simulink library "Byte_Multiplexers_Lib"  (Simulink 8.1)
settings: Solver=ode45  StartTime=0.0  StopTime=10.0  RelTol=1e-3
libraries: commutil2 x35, Bit_Multiplexers_Lib x32, Computer_Library x17
settings Model: Creator=uzivatel  LastModifiedBy=uzivatel

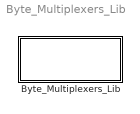
== system Byte_Multiplexers_Lib ==
  Byte_Multiplexers_Lib : Subsystem

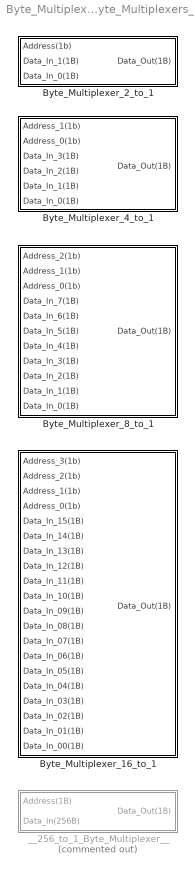
== system Byte_Multiplexers_Lib/Byte_Multiplexers_Lib ==
  Byte_Multiplexer_16_to_1 : Subsystem
  Byte_Multiplexer_2_to_1 : Subsystem
  Byte_Multiplexer_4_to_1 : Subsystem
  Byte_Multiplexer_8_to_1 : Subsystem
  __256_to_1_Byte_Multiplexer__ : Subsystem  Commented=on

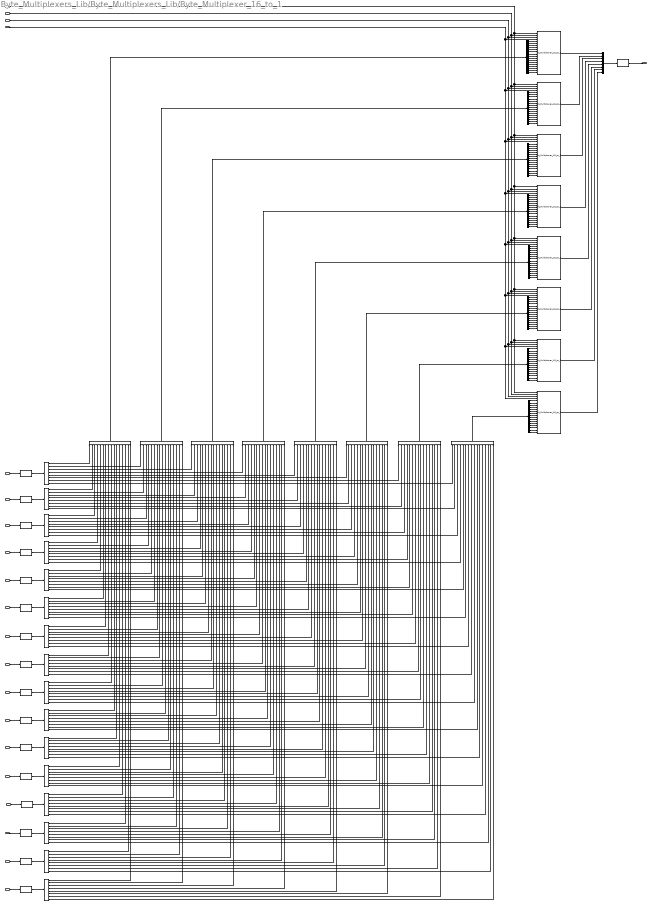
== system Byte_Multiplexers_Lib/Byte_Multiplexers_Lib/Byte_Multiplexer_16_to_1 ==
  Address_3(1b) : Inport
  Address_2(1b) : Inport  Port=2
  Address_1(1b) : Inport  Port=3
  Address_0(1b) : Inport  Port=4
  Data_In_15(1B) : Inport  Port=5
  Data_In_14(1B) : Inport  Port=6
  Data_In_13(1B) : Inport  Port=7
  Data_In_12(1B) : Inport  Port=8
  Data_In_11(1B) : Inport  Port=9
  Data_In_10(1B) : Inport  Port=10
  Data_In_09(1B) : Inport  Port=11
  Data_In_08(1B) : Inport  Port=12
  Data_In_07(1B) : Inport  Port=13
  Data_In_06(1B) : Inport  Port=14
  Data_In_05(1B) : Inport  Port=15
  Data_In_04(1B) : Inport  Port=16
  Data_In_03(1B) : Inport  Port=17
  Data_In_02(1B) : Inport  Port=18
  Data_In_01(1B) : Inport  Port=19
  Data_In_00(1B) : Inport  Port=20
  Bit to Integer Converter1 : commutil2/Bit to Integer Converter  nbits=8  bitOrder=MSB first  signedOutputValues=Unsigned  outDtype=uint8  outDtypeSigned=Inherit via internal rule
  Bit_{0..7} (8 alike) : Mux  Inputs=16
  Bit_Multiplexer_16_to_1(Bit_0) : Bit_Multiplexers_Lib/Bit_Multiplexers_Lib/Bit_Multiplexer_16_to_1
  Bit_Multiplexer_16_to_1(Bit_1) : Bit_Multiplexers_Lib/Bit_Multiplexers_Lib/Bit_Multiplexer_16_to_1
  Bit_Multiplexer_16_to_1(Bit_2) : Bit_Multiplexers_Lib/Bit_Multiplexers_Lib/Bit_Multiplexer_16_to_1
  Bit_Multiplexer_16_to_1(Bit_3) : Bit_Multiplexers_Lib/Bit_Multiplexers_Lib/Bit_Multiplexer_16_to_1
  Bit_Multiplexer_16_to_1(Bit_4) : Bit_Multiplexers_Lib/Bit_Multiplexers_Lib/Bit_Multiplexer_16_to_1
  Bit_Multiplexer_16_to_1(Bit_5) : Bit_Multiplexers_Lib/Bit_Multiplexers_Lib/Bit_Multiplexer_16_to_1
  Bit_Multiplexer_16_to_1(Bit_6) : Bit_Multiplexers_Lib/Bit_Multiplexers_Lib/Bit_Multiplexer_16_to_1
  Bit_Multiplexer_16_to_1(Bit_7) : Bit_Multiplexers_Lib/Bit_Multiplexers_Lib/Bit_Multiplexer_16_to_1
  Byte_{0..15} (16 alike) : Demux  Outputs=8
  Demux{,1..7} (8 alike) : Demux  Outputs=16
  Integer to Bit Converter{1..16} (16 alike) : commutil2/Integer to Bit Converter  nbits=8  signedInputValues=Unsigned  bitOrder=MSB first  outDtype=boolean
  Mux : Mux  Inputs=8
  Data_Out(1B) : Outport
  wires:
  Integer to Bit Converter7/1 -> Byte_15/1
  Data_In_15(1B)/1 -> Integer to Bit Converter7/1
  Mux/1 -> Bit to Integer Converter1/1
  Bit to Integer Converter1/1 -> Data_Out(1B)/1
  Bit_0/1 -> Demux7/1
  Bit_1/1 -> Demux6/1
  Bit_2/1 -> Demux5/1
  Bit_3/1 -> Demux4/1
  Bit_4/1 -> Demux3/1
  Bit_5/1 -> Demux2/1
  Bit_6/1 -> Demux1/1
  Bit_7/1 -> Demux/1
  Byte_9/8 -> Bit_0/7
  Byte_7/7 -> Bit_1/9
  Byte_8/1 -> Bit_7/8
  Byte_9/1 -> Bit_7/7
  Byte_10/1 -> Bit_7/6
  Byte_11/1 -> Bit_7/5
  Byte_12/1 -> Bit_7/4
  Byte_13/1 -> Bit_7/3
  Byte_14/1 -> Bit_7/2
  Address_0(1b)/1 -> Bit_Multiplexer_16_to_1(Bit_5)/4, Bit_Multiplexer_16_to_1(Bit_0)/4, Bit_Multiplexer_16_to_1(Bit_1)/4, Bit_Multiplexer_16_to_1(Bit_2)/4, Bit_Multiplexer_16_to_1(Bit_3)/4, Bit_Multiplexer_16_to_1(Bit_4)/4, Bit_Multiplexer_16_to_1(Bit_6)/4, Bit_Multiplexer_16_to_1(Bit_7)/4
  Address_1(1b)/1 -> Bit_Multiplexer_16_to_1(Bit_5)/3, Bit_Multiplexer_16_to_1(Bit_0)/3, Bit_Multiplexer_16_to_1(Bit_1)/3, Bit_Multiplexer_16_to_1(Bit_2)/3, Bit_Multiplexer_16_to_1(Bit_3)/3, Bit_Multiplexer_16_to_1(Bit_4)/3, Bit_Multiplexer_16_to_1(Bit_6)/3, Bit_Multiplexer_16_to_1(Bit_7)/3
  Address_2(1b)/1 -> Bit_Multiplexer_16_to_1(Bit_6)/2, Bit_Multiplexer_16_to_1(Bit_5)/2, Bit_Multiplexer_16_to_1(Bit_4)/2, Bit_Multiplexer_16_to_1(Bit_2)/2, Bit_Multiplexer_16_to_1(Bit_0)/2, Bit_Multiplexer_16_to_1(Bit_1)/2, Bit_Multiplexer_16_to_1(Bit_3)/2, Bit_Multiplexer_16_to_1(Bit_7)/2
  Address_3(1b)/1 -> Bit_Multiplexer_16_to_1(Bit_5)/1, Bit_Multiplexer_16_to_1(Bit_0)/1, Bit_Multiplexer_16_to_1(Bit_1)/1, Bit_Multiplexer_16_to_1(Bit_2)/1, Bit_Multiplexer_16_to_1(Bit_3)/1, Bit_Multiplexer_16_to_1(Bit_4)/1, Bit_Multiplexer_16_to_1(Bit_6)/1, Bit_Multiplexer_16_to_1(Bit_7)/1
  Bit_Multiplexer_16_to_1(Bit_4)/1 -> Mux/4
  Bit_Multiplexer_16_to_1(Bit_5)/1 -> Mux/3
  Bit_Multiplexer_16_to_1(Bit_6)/1 -> Mux/2
  Bit_Multiplexer_16_to_1(Bit_7)/1 -> Mux/1
  Bit_Multiplexer_16_to_1(Bit_3)/1 -> Mux/5
  Bit_Multiplexer_16_to_1(Bit_2)/1 -> Mux/6
  Bit_Multiplexer_16_to_1(Bit_1)/1 -> Mux/7
  Bit_Multiplexer_16_to_1(Bit_0)/1 -> Mux/8
  Byte_0/8 -> Bit_0/16
  Byte_1/8 -> Bit_0/15
  Byte_2/8 -> Bit_0/14
  Byte_3/8 -> Bit_0/13
  Byte_4/8 -> Bit_0/12
  Byte_5/8 -> Bit_0/11
  Byte_6/8 -> Bit_0/10
  Byte_7/8 -> Bit_0/9
  Byte_8/8 -> Bit_0/8
  Byte_9/7 -> Bit_1/7
  Byte_10/8 -> Bit_0/6
  Byte_11/8 -> Bit_0/5
  Byte_12/8 -> Bit_0/4
  Byte_13/8 -> Bit_0/3
  Byte_14/8 -> Bit_0/2
  Byte_15/8 -> Bit_0/1
  Byte_0/7 -> Bit_1/16
  Byte_1/7 -> Bit_1/15
  Byte_2/7 -> Bit_1/14
  Byte_3/7 -> Bit_1/13
  Byte_4/7 -> Bit_1/12
  Byte_5/7 -> Bit_1/11
  Byte_6/7 -> Bit_1/10
  Byte_8/7 -> Bit_1/8
  Byte_10/7 -> Bit_1/6
  Byte_11/7 -> Bit_1/5
  Byte_12/7 -> Bit_1/4
  Byte_13/7 -> Bit_1/3
  Byte_14/7 -> Bit_1/2
  Byte_15/7 -> Bit_1/1
  Byte_0/6 -> Bit_2/16
  Byte_1/6 -> Bit_2/15
  Byte_2/6 -> Bit_2/14
  Byte_3/6 -> Bit_2/13
  Byte_4/6 -> Bit_2/12
  Byte_5/6 -> Bit_2/11
  Byte_6/6 -> Bit_2/10
  Byte_7/6 -> Bit_2/9
  Byte_8/6 -> Bit_2/8
  Byte_9/6 -> Bit_2/7
  Byte_10/6 -> Bit_2/6
  Byte_11/6 -> Bit_2/5
  Byte_12/6 -> Bit_2/4
  Byte_13/6 -> Bit_2/3
  Byte_14/6 -> Bit_2/2
  Byte_15/6 -> Bit_2/1
  Byte_0/5 -> Bit_3/16
  Byte_1/5 -> Bit_3/15
  Byte_2/5 -> Bit_3/14
  Byte_3/5 -> Bit_3/13
  Byte_4/5 -> Bit_3/12
  Byte_5/5 -> Bit_3/11
  Byte_6/5 -> Bit_3/10
  Byte_7/5 -> Bit_3/9
  Byte_8/5 -> Bit_3/8
  Byte_9/5 -> Bit_3/7
  Byte_10/5 -> Bit_3/6
  Byte_11/5 -> Bit_3/5
  Byte_12/5 -> Bit_3/4
  Byte_13/5 -> Bit_3/3
  Byte_14/5 -> Bit_3/2
  Byte_15/5 -> Bit_3/1
  Byte_0/4 -> Bit_4/16
  Byte_1/4 -> Bit_4/15
  Byte_2/4 -> Bit_4/14
  Byte_3/4 -> Bit_4/13
  Byte_4/4 -> Bit_4/12
  Byte_5/4 -> Bit_4/11
  Byte_6/4 -> Bit_4/10
  Byte_7/4 -> Bit_4/9
  Byte_8/4 -> Bit_4/8
  Byte_9/4 -> Bit_4/7
  Byte_10/4 -> Bit_4/6
  Byte_11/4 -> Bit_4/5
  Byte_12/4 -> Bit_4/4
  Byte_13/4 -> Bit_4/3
  Byte_14/4 -> Bit_4/2
  Byte_15/4 -> Bit_4/1
  Byte_0/3 -> Bit_5/16
  Byte_1/3 -> Bit_5/15
  Byte_2/3 -> Bit_5/14
  Byte_3/3 -> Bit_5/13
  Byte_4/3 -> Bit_5/12
  Byte_5/3 -> Bit_5/11
  Byte_6/3 -> Bit_5/10
  Byte_7/3 -> Bit_5/9
  Byte_8/3 -> Bit_5/8
  Byte_9/3 -> Bit_5/7
  Byte_10/3 -> Bit_5/6
  Byte_11/3 -> Bit_5/5
  Byte_12/3 -> Bit_5/4
  Byte_13/3 -> Bit_5/3
  Byte_14/3 -> Bit_5/2
  Byte_15/3 -> Bit_5/1
  Byte_0/2 -> Bit_6/16
  Byte_1/2 -> Bit_6/15
  Byte_2/2 -> Bit_6/14
  Byte_3/2 -> Bit_6/13
  Byte_4/2 -> Bit_6/12
  Byte_5/2 -> Bit_6/11
  Byte_6/2 -> Bit_6/10
  Byte_7/2 -> Bit_6/9
  Byte_8/2 -> Bit_6/8
  Byte_9/2 -> Bit_6/7
  Byte_10/2 -> Bit_6/6
  Byte_11/2 -> Bit_6/5
  Byte_12/2 -> Bit_6/4
  Byte_13/2 -> Bit_6/3
  Byte_14/2 -> Bit_6/2
  Byte_15/2 -> Bit_6/1
  Byte_0/1 -> Bit_7/16
  Byte_1/1 -> Bit_7/15
  Byte_2/1 -> Bit_7/14
  Byte_3/1 -> Bit_7/13
  Byte_4/1 -> Bit_7/12
  Byte_5/1 -> Bit_7/11
  Byte_6/1 -> Bit_7/10
  Byte_7/1 -> Bit_7/9
  Byte_15/1 -> Bit_7/1
  Integer to Bit Converter1/1 -> Byte_14/1
  Data_In_14(1B)/1 -> Integer to Bit Converter1/1
  Integer to Bit Converter2/1 -> Byte_13/1
  Data_In_13(1B)/1 -> Integer to Bit Converter2/1
  Integer to Bit Converter3/1 -> Byte_12/1
  Data_In_12(1B)/1 -> Integer to Bit Converter3/1
  Integer to Bit Converter4/1 -> Byte_11/1
  Data_In_11(1B)/1 -> Integer to Bit Converter4/1
  Integer to Bit Converter5/1 -> Byte_10/1
  Data_In_10(1B)/1 -> Integer to Bit Converter5/1
  Integer to Bit Converter6/1 -> Byte_9/1
  Data_In_09(1B)/1 -> Integer to Bit Converter6/1
  Integer to Bit Converter8/1 -> Byte_8/1
  Data_In_08(1B)/1 -> Integer to Bit Converter8/1
  Integer to Bit Converter9/1 -> Byte_7/1
  Data_In_07(1B)/1 -> Integer to Bit Converter9/1
  Integer to Bit Converter10/1 -> Byte_6/1
  Data_In_06(1B)/1 -> Integer to Bit Converter10/1
  Integer to Bit Converter11/1 -> Byte_5/1
  Data_In_05(1B)/1 -> Integer to Bit Converter11/1
  Integer to Bit Converter12/1 -> Byte_4/1
  Data_In_04(1B)/1 -> Integer to Bit Converter12/1
  Integer to Bit Converter13/1 -> Byte_3/1
  Data_In_03(1B)/1 -> Integer to Bit Converter13/1
  Integer to Bit Converter14/1 -> Byte_2/1
  Data_In_02(1B)/1 -> Integer to Bit Converter14/1
  Integer to Bit Converter15/1 -> Byte_1/1
  Data_In_01(1B)/1 -> Integer to Bit Converter15/1
  Integer to Bit Converter16/1 -> Byte_0/1
  Data_In_00(1B)/1 -> Integer to Bit Converter16/1
  Demux/1 -> Bit_Multiplexer_16_to_1(Bit_7)/5
  Demux/2 -> Bit_Multiplexer_16_to_1(Bit_7)/6
  Demux/3 -> Bit_Multiplexer_16_to_1(Bit_7)/7
  Demux/4 -> Bit_Multiplexer_16_to_1(Bit_7)/8
  Demux/5 -> Bit_Multiplexer_16_to_1(Bit_7)/9
  Demux/6 -> Bit_Multiplexer_16_to_1(Bit_7)/10
  Demux/7 -> Bit_Multiplexer_16_to_1(Bit_7)/11
  Demux/8 -> Bit_Multiplexer_16_to_1(Bit_7)/12
  Demux/9 -> Bit_Multiplexer_16_to_1(Bit_7)/13
  Demux/10 -> Bit_Multiplexer_16_to_1(Bit_7)/14
  Demux/11 -> Bit_Multiplexer_16_to_1(Bit_7)/15
  Demux/12 -> Bit_Multiplexer_16_to_1(Bit_7)/16
  Demux/13 -> Bit_Multiplexer_16_to_1(Bit_7)/17
  Demux/14 -> Bit_Multiplexer_16_to_1(Bit_7)/18
  Demux/15 -> Bit_Multiplexer_16_to_1(Bit_7)/19
  Demux/16 -> Bit_Multiplexer_16_to_1(Bit_7)/20
  Demux1/1 -> Bit_Multiplexer_16_to_1(Bit_6)/5
  Demux1/2 -> Bit_Multiplexer_16_to_1(Bit_6)/6
  Demux1/3 -> Bit_Multiplexer_16_to_1(Bit_6)/7
  Demux1/4 -> Bit_Multiplexer_16_to_1(Bit_6)/8
  Demux1/5 -> Bit_Multiplexer_16_to_1(Bit_6)/9
  Demux1/6 -> Bit_Multiplexer_16_to_1(Bit_6)/10
  Demux1/7 -> Bit_Multiplexer_16_to_1(Bit_6)/11
  Demux1/8 -> Bit_Multiplexer_16_to_1(Bit_6)/12
  Demux1/9 -> Bit_Multiplexer_16_to_1(Bit_6)/13
  Demux1/10 -> Bit_Multiplexer_16_to_1(Bit_6)/14
  Demux1/11 -> Bit_Multiplexer_16_to_1(Bit_6)/15
  Demux1/12 -> Bit_Multiplexer_16_to_1(Bit_6)/16
  Demux1/13 -> Bit_Multiplexer_16_to_1(Bit_6)/17
  Demux1/14 -> Bit_Multiplexer_16_to_1(Bit_6)/18
  Demux1/15 -> Bit_Multiplexer_16_to_1(Bit_6)/19
  Demux1/16 -> Bit_Multiplexer_16_to_1(Bit_6)/20
  Demux2/1 -> Bit_Multiplexer_16_to_1(Bit_5)/5
  Demux2/2 -> Bit_Multiplexer_16_to_1(Bit_5)/6
  Demux2/3 -> Bit_Multiplexer_16_to_1(Bit_5)/7
  Demux2/4 -> Bit_Multiplexer_16_to_1(Bit_5)/8
  Demux2/5 -> Bit_Multiplexer_16_to_1(Bit_5)/9
  Demux2/6 -> Bit_Multiplexer_16_to_1(Bit_5)/10
  Demux2/7 -> Bit_Multiplexer_16_to_1(Bit_5)/11
  Demux2/8 -> Bit_Multiplexer_16_to_1(Bit_5)/12
  Demux2/9 -> Bit_Multiplexer_16_to_1(Bit_5)/13
  Demux2/10 -> Bit_Multiplexer_16_to_1(Bit_5)/14
  Demux2/11 -> Bit_Multiplexer_16_to_1(Bit_5)/15
  Demux2/12 -> Bit_Multiplexer_16_to_1(Bit_5)/16
  Demux2/13 -> Bit_Multiplexer_16_to_1(Bit_5)/17
  Demux2/14 -> Bit_Multiplexer_16_to_1(Bit_5)/18
  Demux2/15 -> Bit_Multiplexer_16_to_1(Bit_5)/19
  Demux2/16 -> Bit_Multiplexer_16_to_1(Bit_5)/20
  Demux3/1 -> Bit_Multiplexer_16_to_1(Bit_4)/5
  Demux3/2 -> Bit_Multiplexer_16_to_1(Bit_4)/6
  Demux3/3 -> Bit_Multiplexer_16_to_1(Bit_4)/7
  Demux3/4 -> Bit_Multiplexer_16_to_1(Bit_4)/8
  Demux3/5 -> Bit_Multiplexer_16_to_1(Bit_4)/9
  Demux3/6 -> Bit_Multiplexer_16_to_1(Bit_4)/10
  Demux3/7 -> Bit_Multiplexer_16_to_1(Bit_4)/11
  Demux3/8 -> Bit_Multiplexer_16_to_1(Bit_4)/12
  Demux3/9 -> Bit_Multiplexer_16_to_1(Bit_4)/13
  Demux3/10 -> Bit_Multiplexer_16_to_1(Bit_4)/14
  Demux3/11 -> Bit_Multiplexer_16_to_1(Bit_4)/15
  Demux3/12 -> Bit_Multiplexer_16_to_1(Bit_4)/16
  Demux3/13 -> Bit_Multiplexer_16_to_1(Bit_4)/17
  Demux3/14 -> Bit_Multiplexer_16_to_1(Bit_4)/18
  Demux3/15 -> Bit_Multiplexer_16_to_1(Bit_4)/19
  Demux3/16 -> Bit_Multiplexer_16_to_1(Bit_4)/20
  Demux4/1 -> Bit_Multiplexer_16_to_1(Bit_3)/5
  Demux4/2 -> Bit_Multiplexer_16_to_1(Bit_3)/6
  Demux4/3 -> Bit_Multiplexer_16_to_1(Bit_3)/7
  Demux4/4 -> Bit_Multiplexer_16_to_1(Bit_3)/8
  Demux4/5 -> Bit_Multiplexer_16_to_1(Bit_3)/9
  Demux4/6 -> Bit_Multiplexer_16_to_1(Bit_3)/10
  Demux4/7 -> Bit_Multiplexer_16_to_1(Bit_3)/11
  Demux4/8 -> Bit_Multiplexer_16_to_1(Bit_3)/12
  Demux4/9 -> Bit_Multiplexer_16_to_1(Bit_3)/13
  Demux4/10 -> Bit_Multiplexer_16_to_1(Bit_3)/14
  Demux4/11 -> Bit_Multiplexer_16_to_1(Bit_3)/15
  Demux4/12 -> Bit_Multiplexer_16_to_1(Bit_3)/16
  Demux4/13 -> Bit_Multiplexer_16_to_1(Bit_3)/17
  Demux4/14 -> Bit_Multiplexer_16_to_1(Bit_3)/18
  Demux4/15 -> Bit_Multiplexer_16_to_1(Bit_3)/19
  Demux4/16 -> Bit_Multiplexer_16_to_1(Bit_3)/20
  Demux5/1 -> Bit_Multiplexer_16_to_1(Bit_2)/5
  Demux5/2 -> Bit_Multiplexer_16_to_1(Bit_2)/6
  Demux5/3 -> Bit_Multiplexer_16_to_1(Bit_2)/7
  Demux5/4 -> Bit_Multiplexer_16_to_1(Bit_2)/8
  Demux5/5 -> Bit_Multiplexer_16_to_1(Bit_2)/9
  Demux5/6 -> Bit_Multiplexer_16_to_1(Bit_2)/10
  Demux5/7 -> Bit_Multiplexer_16_to_1(Bit_2)/11
  Demux5/8 -> Bit_Multiplexer_16_to_1(Bit_2)/12
  Demux5/9 -> Bit_Multiplexer_16_to_1(Bit_2)/13
  Demux5/10 -> Bit_Multiplexer_16_to_1(Bit_2)/14
  Demux5/11 -> Bit_Multiplexer_16_to_1(Bit_2)/15
  Demux5/12 -> Bit_Multiplexer_16_to_1(Bit_2)/16
  Demux5/13 -> Bit_Multiplexer_16_to_1(Bit_2)/17
  Demux5/14 -> Bit_Multiplexer_16_to_1(Bit_2)/18
  Demux5/15 -> Bit_Multiplexer_16_to_1(Bit_2)/19
  Demux5/16 -> Bit_Multiplexer_16_to_1(Bit_2)/20
  Demux6/1 -> Bit_Multiplexer_16_to_1(Bit_1)/5
  Demux6/2 -> Bit_Multiplexer_16_to_1(Bit_1)/6
  Demux6/3 -> Bit_Multiplexer_16_to_1(Bit_1)/7
  Demux6/4 -> Bit_Multiplexer_16_to_1(Bit_1)/8
  Demux6/5 -> Bit_Multiplexer_16_to_1(Bit_1)/9
  Demux6/6 -> Bit_Multiplexer_16_to_1(Bit_1)/10
  Demux6/7 -> Bit_Multiplexer_16_to_1(Bit_1)/11
  Demux6/8 -> Bit_Multiplexer_16_to_1(Bit_1)/12
  Demux6/9 -> Bit_Multiplexer_16_to_1(Bit_1)/13
  Demux6/10 -> Bit_Multiplexer_16_to_1(Bit_1)/14
  Demux6/11 -> Bit_Multiplexer_16_to_1(Bit_1)/15
  Demux6/12 -> Bit_Multiplexer_16_to_1(Bit_1)/16
  Demux6/13 -> Bit_Multiplexer_16_to_1(Bit_1)/17
  Demux6/14 -> Bit_Multiplexer_16_to_1(Bit_1)/18
  Demux6/15 -> Bit_Multiplexer_16_to_1(Bit_1)/19
  Demux6/16 -> Bit_Multiplexer_16_to_1(Bit_1)/20
  Demux7/1 -> Bit_Multiplexer_16_to_1(Bit_0)/5
  Demux7/2 -> Bit_Multiplexer_16_to_1(Bit_0)/6
  Demux7/3 -> Bit_Multiplexer_16_to_1(Bit_0)/7
  Demux7/4 -> Bit_Multiplexer_16_to_1(Bit_0)/8
  Demux7/5 -> Bit_Multiplexer_16_to_1(Bit_0)/9
  Demux7/6 -> Bit_Multiplexer_16_to_1(Bit_0)/10
  Demux7/7 -> Bit_Multiplexer_16_to_1(Bit_0)/11
  Demux7/8 -> Bit_Multiplexer_16_to_1(Bit_0)/12
  Demux7/9 -> Bit_Multiplexer_16_to_1(Bit_0)/13
  Demux7/10 -> Bit_Multiplexer_16_to_1(Bit_0)/14
  Demux7/11 -> Bit_Multiplexer_16_to_1(Bit_0)/15
  Demux7/12 -> Bit_Multiplexer_16_to_1(Bit_0)/16
  Demux7/13 -> Bit_Multiplexer_16_to_1(Bit_0)/17
  Demux7/14 -> Bit_Multiplexer_16_to_1(Bit_0)/18
  Demux7/15 -> Bit_Multiplexer_16_to_1(Bit_0)/19
  Demux7/16 -> Bit_Multiplexer_16_to_1(Bit_0)/20

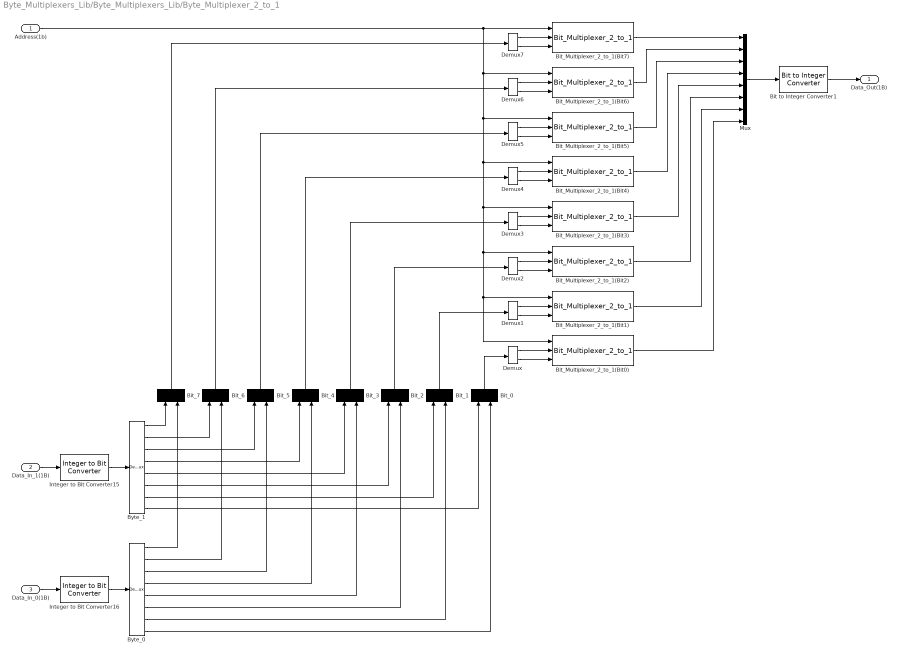
== system Byte_Multiplexers_Lib/Byte_Multiplexers_Lib/Byte_Multiplexer_2_to_1 ==
  Address(1b) : Inport
  Data_In_1(1B) : Inport  Port=2
  Data_In_0(1B) : Inport  Port=3
  Bit to Integer Converter1 : commutil2/Bit to Integer Converter  nbits=8  bitOrder=MSB first  signedOutputValues=Unsigned  outDtype=uint8  outDtypeSigned=Inherit via internal rule
  Bit_{0..7} (8 alike) : Mux  Inputs=2
  Bit_Multiplexer_2_to_1(Bit0) : Bit_Multiplexers_Lib/Bit_Multiplexers_Lib/Bit_Multiplexer_2_to_1
  Bit_Multiplexer_2_to_1(Bit1) : Bit_Multiplexers_Lib/Bit_Multiplexers_Lib/Bit_Multiplexer_2_to_1
  Bit_Multiplexer_2_to_1(Bit2) : Bit_Multiplexers_Lib/Bit_Multiplexers_Lib/Bit_Multiplexer_2_to_1
  Bit_Multiplexer_2_to_1(Bit3) : Bit_Multiplexers_Lib/Bit_Multiplexers_Lib/Bit_Multiplexer_2_to_1
  Bit_Multiplexer_2_to_1(Bit4) : Bit_Multiplexers_Lib/Bit_Multiplexers_Lib/Bit_Multiplexer_2_to_1
  Bit_Multiplexer_2_to_1(Bit5) : Bit_Multiplexers_Lib/Bit_Multiplexers_Lib/Bit_Multiplexer_2_to_1
  Bit_Multiplexer_2_to_1(Bit6) : Bit_Multiplexers_Lib/Bit_Multiplexers_Lib/Bit_Multiplexer_2_to_1
  Bit_Multiplexer_2_to_1(Bit7) : Bit_Multiplexers_Lib/Bit_Multiplexers_Lib/Bit_Multiplexer_2_to_1
  Byte_0 : Demux  Outputs=8
  Byte_1 : Demux  Outputs=8
  Demux{,1..7} (8 alike) : Demux  Outputs=2
  Integer to Bit Converter15 : commutil2/Integer to Bit Converter  nbits=8  signedInputValues=Unsigned  bitOrder=MSB first  outDtype=boolean
  Integer to Bit Converter16 : commutil2/Integer to Bit Converter  nbits=8  signedInputValues=Unsigned  bitOrder=MSB first  outDtype=boolean
  Mux : Mux  Inputs=8
  Data_Out(1B) : Outport
  wires:
  Mux/1 -> Bit to Integer Converter1/1
  Bit to Integer Converter1/1 -> Data_Out(1B)/1
  Bit_0/1 -> Demux/1
  Bit_1/1 -> Demux1/1
  Bit_2/1 -> Demux2/1
  Bit_3/1 -> Demux3/1
  Bit_4/1 -> Demux4/1
  Bit_5/1 -> Demux5/1
  Bit_6/1 -> Demux6/1
  Bit_7/1 -> Demux7/1
  Address(1b)/1 -> Bit_Multiplexer_2_to_1(Bit7)/1, Bit_Multiplexer_2_to_1(Bit0)/1, Bit_Multiplexer_2_to_1(Bit1)/1, Bit_Multiplexer_2_to_1(Bit2)/1, Bit_Multiplexer_2_to_1(Bit3)/1, Bit_Multiplexer_2_to_1(Bit4)/1, Bit_Multiplexer_2_to_1(Bit5)/1, Bit_Multiplexer_2_to_1(Bit6)/1
  Bit_Multiplexer_2_to_1(Bit4)/1 -> Mux/4
  Bit_Multiplexer_2_to_1(Bit5)/1 -> Mux/3
  Bit_Multiplexer_2_to_1(Bit6)/1 -> Mux/2
  Bit_Multiplexer_2_to_1(Bit7)/1 -> Mux/1
  Bit_Multiplexer_2_to_1(Bit3)/1 -> Mux/5
  Bit_Multiplexer_2_to_1(Bit2)/1 -> Mux/6
  Bit_Multiplexer_2_to_1(Bit1)/1 -> Mux/7
  Bit_Multiplexer_2_to_1(Bit0)/1 -> Mux/8
  Byte_0/8 -> Bit_0/2
  Byte_1/8 -> Bit_0/1
  Byte_0/7 -> Bit_1/2
  Byte_1/7 -> Bit_1/1
  Byte_0/6 -> Bit_2/2
  Byte_1/6 -> Bit_2/1
  Byte_0/5 -> Bit_3/2
  Byte_1/5 -> Bit_3/1
  Byte_0/4 -> Bit_4/2
  Byte_1/4 -> Bit_4/1
  Byte_0/3 -> Bit_5/2
  Byte_1/3 -> Bit_5/1
  Byte_0/2 -> Bit_6/2
  Byte_1/2 -> Bit_6/1
  Byte_0/1 -> Bit_7/2
  Byte_1/1 -> Bit_7/1
  Integer to Bit Converter15/1 -> Byte_1/1
  Data_In_1(1B)/1 -> Integer to Bit Converter15/1
  Integer to Bit Converter16/1 -> Byte_0/1
  Data_In_0(1B)/1 -> Integer to Bit Converter16/1
  Demux/1 -> Bit_Multiplexer_2_to_1(Bit0)/2
  Demux/2 -> Bit_Multiplexer_2_to_1(Bit0)/3
  Demux1/1 -> Bit_Multiplexer_2_to_1(Bit1)/2
  Demux1/2 -> Bit_Multiplexer_2_to_1(Bit1)/3
  Demux2/1 -> Bit_Multiplexer_2_to_1(Bit2)/2
  Demux2/2 -> Bit_Multiplexer_2_to_1(Bit2)/3
  Demux3/2 -> Bit_Multiplexer_2_to_1(Bit3)/3
  Demux3/1 -> Bit_Multiplexer_2_to_1(Bit3)/2
  Demux4/2 -> Bit_Multiplexer_2_to_1(Bit4)/3
  Demux4/1 -> Bit_Multiplexer_2_to_1(Bit4)/2
  Demux5/1 -> Bit_Multiplexer_2_to_1(Bit5)/2
  Demux5/2 -> Bit_Multiplexer_2_to_1(Bit5)/3
  Demux6/1 -> Bit_Multiplexer_2_to_1(Bit6)/2
  Demux6/2 -> Bit_Multiplexer_2_to_1(Bit6)/3
  Demux7/2 -> Bit_Multiplexer_2_to_1(Bit7)/3
  Demux7/1 -> Bit_Multiplexer_2_to_1(Bit7)/2

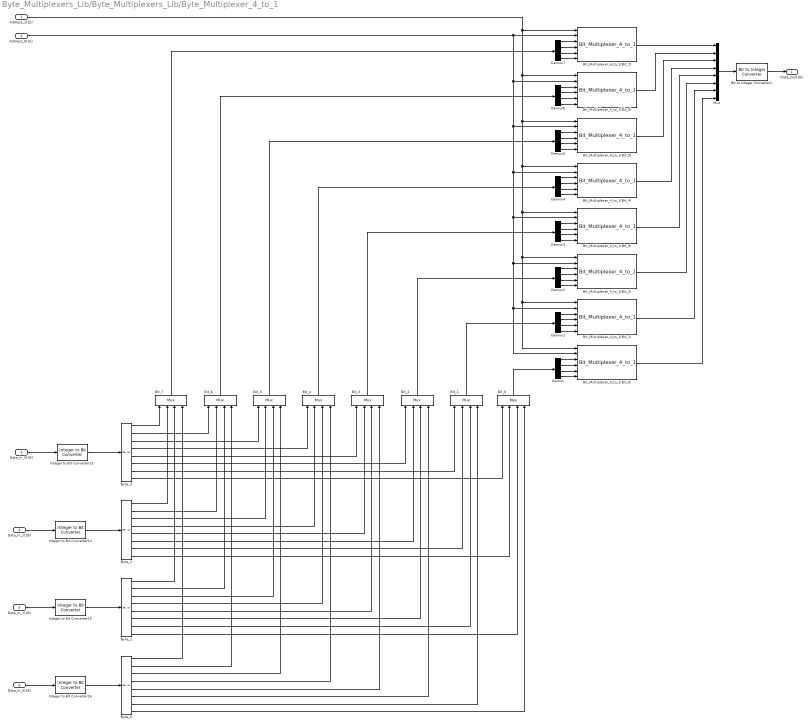
== system Byte_Multiplexers_Lib/Byte_Multiplexers_Lib/Byte_Multiplexer_4_to_1 ==
  Address_1(1b) : Inport
  Address_0(1b) : Inport  Port=2
  Data_In_3(1B) : Inport  Port=3
  Data_In_2(1B) : Inport  Port=4
  Data_In_1(1B) : Inport  Port=5
  Data_In_0(1B) : Inport  Port=6
  Bit to Integer Converter1 : commutil2/Bit to Integer Converter  nbits=8  bitOrder=MSB first  signedOutputValues=Unsigned  outDtype=uint8  outDtypeSigned=Inherit via internal rule
  Bit_{0..7} (8 alike) : Mux
  Bit_Multiplexer_4_to_1(Bit_0) : Bit_Multiplexers_Lib/Bit_Multiplexers_Lib/Bit_Multiplexer_4_to_1
  Bit_Multiplexer_4_to_1(Bit_1) : Bit_Multiplexers_Lib/Bit_Multiplexers_Lib/Bit_Multiplexer_4_to_1
  Bit_Multiplexer_4_to_1(Bit_2) : Bit_Multiplexers_Lib/Bit_Multiplexers_Lib/Bit_Multiplexer_4_to_1
  Bit_Multiplexer_4_to_1(Bit_3) : Bit_Multiplexers_Lib/Bit_Multiplexers_Lib/Bit_Multiplexer_4_to_1
  Bit_Multiplexer_4_to_1(Bit_4) : Bit_Multiplexers_Lib/Bit_Multiplexers_Lib/Bit_Multiplexer_4_to_1
  Bit_Multiplexer_4_to_1(Bit_5) : Bit_Multiplexers_Lib/Bit_Multiplexers_Lib/Bit_Multiplexer_4_to_1
  Bit_Multiplexer_4_to_1(Bit_6) : Bit_Multiplexers_Lib/Bit_Multiplexers_Lib/Bit_Multiplexer_4_to_1
  Bit_Multiplexer_4_to_1(Bit_7) : Bit_Multiplexers_Lib/Bit_Multiplexers_Lib/Bit_Multiplexer_4_to_1
  Byte_{0..3} (4 alike) : Demux  Outputs=8
  Demux{,1..7} (8 alike) : Demux
  Integer to Bit Converter{13..16} (4 alike) : commutil2/Integer to Bit Converter  nbits=8  signedInputValues=Unsigned  bitOrder=MSB first  outDtype=boolean
  Mux : Mux  Inputs=8
  Data_Out(1B) : Outport
  wires:
  Mux/1 -> Bit to Integer Converter1/1
  Bit to Integer Converter1/1 -> Data_Out(1B)/1
  Bit_0/1 -> Demux/1
  Bit_1/1 -> Demux1/1
  Bit_2/1 -> Demux2/1
  Bit_3/1 -> Demux3/1
  Bit_4/1 -> Demux4/1
  Bit_5/1 -> Demux5/1
  Bit_6/1 -> Demux6/1
  Bit_7/1 -> Demux7/1
  Address_0(1b)/1 -> Bit_Multiplexer_4_to_1(Bit_7)/2, Bit_Multiplexer_4_to_1(Bit_0)/2, Bit_Multiplexer_4_to_1(Bit_1)/2, Bit_Multiplexer_4_to_1(Bit_2)/2, Bit_Multiplexer_4_to_1(Bit_3)/2, Bit_Multiplexer_4_to_1(Bit_4)/2, Bit_Multiplexer_4_to_1(Bit_5)/2, Bit_Multiplexer_4_to_1(Bit_6)/2
  Address_1(1b)/1 -> Bit_Multiplexer_4_to_1(Bit_7)/1, Bit_Multiplexer_4_to_1(Bit_0)/1, Bit_Multiplexer_4_to_1(Bit_1)/1, Bit_Multiplexer_4_to_1(Bit_2)/1, Bit_Multiplexer_4_to_1(Bit_3)/1, Bit_Multiplexer_4_to_1(Bit_4)/1, Bit_Multiplexer_4_to_1(Bit_5)/1, Bit_Multiplexer_4_to_1(Bit_6)/1
  Bit_Multiplexer_4_to_1(Bit_4)/1 -> Mux/4
  Bit_Multiplexer_4_to_1(Bit_5)/1 -> Mux/3
  Bit_Multiplexer_4_to_1(Bit_6)/1 -> Mux/2
  Bit_Multiplexer_4_to_1(Bit_7)/1 -> Mux/1
  Bit_Multiplexer_4_to_1(Bit_3)/1 -> Mux/5
  Bit_Multiplexer_4_to_1(Bit_2)/1 -> Mux/6
  Bit_Multiplexer_4_to_1(Bit_1)/1 -> Mux/7
  Bit_Multiplexer_4_to_1(Bit_0)/1 -> Mux/8
  Byte_0/8 -> Bit_0/4
  Byte_1/8 -> Bit_0/3
  Byte_2/8 -> Bit_0/2
  Byte_3/8 -> Bit_0/1
  Byte_0/7 -> Bit_1/4
  Byte_1/7 -> Bit_1/3
  Byte_2/7 -> Bit_1/2
  Byte_3/7 -> Bit_1/1
  Byte_0/6 -> Bit_2/4
  Byte_1/6 -> Bit_2/3
  Byte_2/6 -> Bit_2/2
  Byte_3/6 -> Bit_2/1
  Byte_0/5 -> Bit_3/4
  Byte_1/5 -> Bit_3/3
  Byte_2/5 -> Bit_3/2
  Byte_3/5 -> Bit_3/1
  Byte_0/4 -> Bit_4/4
  Byte_1/4 -> Bit_4/3
  Byte_2/4 -> Bit_4/2
  Byte_3/4 -> Bit_4/1
  Byte_0/3 -> Bit_5/4
  Byte_1/3 -> Bit_5/3
  Byte_2/3 -> Bit_5/2
  Byte_3/3 -> Bit_5/1
  Byte_0/2 -> Bit_6/4
  Byte_1/2 -> Bit_6/3
  Byte_2/2 -> Bit_6/2
  Byte_3/2 -> Bit_6/1
  Byte_0/1 -> Bit_7/4
  Byte_1/1 -> Bit_7/3
  Byte_2/1 -> Bit_7/2
  Byte_3/1 -> Bit_7/1
  Integer to Bit Converter13/1 -> Byte_3/1
  Data_In_3(1B)/1 -> Integer to Bit Converter13/1
  Integer to Bit Converter14/1 -> Byte_2/1
  Data_In_2(1B)/1 -> Integer to Bit Converter14/1
  Integer to Bit Converter15/1 -> Byte_1/1
  Data_In_1(1B)/1 -> Integer to Bit Converter15/1
  Integer to Bit Converter16/1 -> Byte_0/1
  Data_In_0(1B)/1 -> Integer to Bit Converter16/1
  Demux/1 -> Bit_Multiplexer_4_to_1(Bit_0)/3
  Demux/2 -> Bit_Multiplexer_4_to_1(Bit_0)/4
  Demux/3 -> Bit_Multiplexer_4_to_1(Bit_0)/5
  Demux/4 -> Bit_Multiplexer_4_to_1(Bit_0)/6
  Demux1/1 -> Bit_Multiplexer_4_to_1(Bit_1)/3
  Demux1/2 -> Bit_Multiplexer_4_to_1(Bit_1)/4
  Demux1/3 -> Bit_Multiplexer_4_to_1(Bit_1)/5
  Demux1/4 -> Bit_Multiplexer_4_to_1(Bit_1)/6
  Demux2/1 -> Bit_Multiplexer_4_to_1(Bit_2)/3
  Demux2/2 -> Bit_Multiplexer_4_to_1(Bit_2)/4
  Demux2/3 -> Bit_Multiplexer_4_to_1(Bit_2)/5
  Demux2/4 -> Bit_Multiplexer_4_to_1(Bit_2)/6
  Demux3/1 -> Bit_Multiplexer_4_to_1(Bit_3)/3
  Demux3/2 -> Bit_Multiplexer_4_to_1(Bit_3)/4
  Demux3/3 -> Bit_Multiplexer_4_to_1(Bit_3)/5
  Demux3/4 -> Bit_Multiplexer_4_to_1(Bit_3)/6
  Demux4/1 -> Bit_Multiplexer_4_to_1(Bit_4)/3
  Demux4/2 -> Bit_Multiplexer_4_to_1(Bit_4)/4
  Demux4/3 -> Bit_Multiplexer_4_to_1(Bit_4)/5
  Demux4/4 -> Bit_Multiplexer_4_to_1(Bit_4)/6
  Demux5/1 -> Bit_Multiplexer_4_to_1(Bit_5)/3
  Demux5/2 -> Bit_Multiplexer_4_to_1(Bit_5)/4
  Demux5/3 -> Bit_Multiplexer_4_to_1(Bit_5)/5
  Demux5/4 -> Bit_Multiplexer_4_to_1(Bit_5)/6
  Demux6/1 -> Bit_Multiplexer_4_to_1(Bit_6)/3
  Demux6/2 -> Bit_Multiplexer_4_to_1(Bit_6)/4
  Demux6/3 -> Bit_Multiplexer_4_to_1(Bit_6)/5
  Demux6/4 -> Bit_Multiplexer_4_to_1(Bit_6)/6
  Demux7/1 -> Bit_Multiplexer_4_to_1(Bit_7)/3
  Demux7/2 -> Bit_Multiplexer_4_to_1(Bit_7)/4
  Demux7/3 -> Bit_Multiplexer_4_to_1(Bit_7)/5
  Demux7/4 -> Bit_Multiplexer_4_to_1(Bit_7)/6

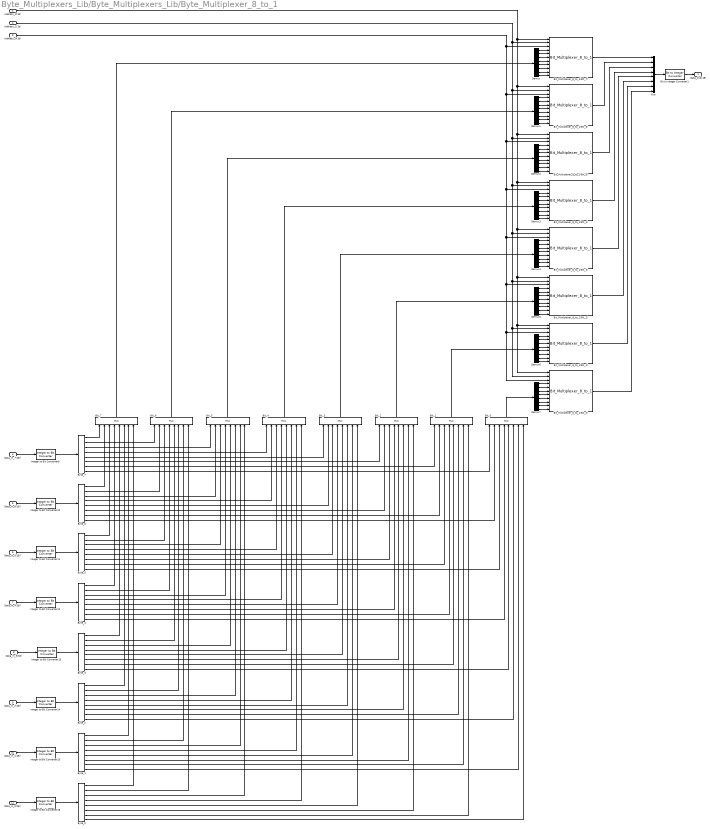
== system Byte_Multiplexers_Lib/Byte_Multiplexers_Lib/Byte_Multiplexer_8_to_1 ==
  Address_2(1b) : Inport
  Address_1(1b) : Inport  Port=2
  Address_0(1b) : Inport  Port=3
  Data_In_7(1B) : Inport  Port=4
  Data_In_6(1B) : Inport  Port=5
  Data_In_5(1B) : Inport  Port=6
  Data_In_4(1B) : Inport  Port=7
  Data_In_3(1B) : Inport  Port=8
  Data_In_2(1B) : Inport  Port=9
  Data_In_1(1B) : Inport  Port=10
  Data_In_0(1B) : Inport  Port=11
  Bit to Integer Converter1 : commutil2/Bit to Integer Converter  nbits=8  bitOrder=MSB first  signedOutputValues=Unsigned  outDtype=uint8  outDtypeSigned=Inherit via internal rule
  Bit_{0..7} (8 alike) : Mux  Inputs=8
  Bit_Multiplexer_8_to_1(Bit_0) : Bit_Multiplexers_Lib/Bit_Multiplexers_Lib/Bit_Multiplexer_8_to_1
  Bit_Multiplexer_8_to_1(Bit_1) : Bit_Multiplexers_Lib/Bit_Multiplexers_Lib/Bit_Multiplexer_8_to_1
  Bit_Multiplexer_8_to_1(Bit_2) : Bit_Multiplexers_Lib/Bit_Multiplexers_Lib/Bit_Multiplexer_8_to_1
  Bit_Multiplexer_8_to_1(Bit_3) : Bit_Multiplexers_Lib/Bit_Multiplexers_Lib/Bit_Multiplexer_8_to_1
  Bit_Multiplexer_8_to_1(Bit_4) : Bit_Multiplexers_Lib/Bit_Multiplexers_Lib/Bit_Multiplexer_8_to_1
  Bit_Multiplexer_8_to_1(Bit_5) : Bit_Multiplexers_Lib/Bit_Multiplexers_Lib/Bit_Multiplexer_8_to_1
  Bit_Multiplexer_8_to_1(Bit_6) : Bit_Multiplexers_Lib/Bit_Multiplexers_Lib/Bit_Multiplexer_8_to_1
  Bit_Multiplexer_8_to_1(Bit_7) : Bit_Multiplexers_Lib/Bit_Multiplexers_Lib/Bit_Multiplexer_8_to_1
  Byte_{0..7} (8 alike) : Demux  Outputs=8
  Demux{,1..7} (8 alike) : Demux  Outputs=8
  Integer to Bit Converter{9..16} (8 alike) : commutil2/Integer to Bit Converter  nbits=8  signedInputValues=Unsigned  bitOrder=MSB first  outDtype=boolean
  Mux : Mux  Inputs=8
  Data_Out(1B) : Outport
  wires:
  Mux/1 -> Bit to Integer Converter1/1
  Bit to Integer Converter1/1 -> Data_Out(1B)/1
  Bit_0/1 -> Demux7/1
  Bit_1/1 -> Demux6/1
  Bit_2/1 -> Demux5/1
  Bit_3/1 -> Demux4/1
  Bit_4/1 -> Demux3/1
  Bit_5/1 -> Demux2/1
  Bit_6/1 -> Demux1/1
  Bit_7/1 -> Demux/1
  Byte_7/7 -> Bit_1/1
  Address_0(1b)/1 -> Bit_Multiplexer_8_to_1(Bit_0)/3, Bit_Multiplexer_8_to_1(Bit_1)/3, Bit_Multiplexer_8_to_1(Bit_2)/3, Bit_Multiplexer_8_to_1(Bit_3)/3, Bit_Multiplexer_8_to_1(Bit_4)/3, Bit_Multiplexer_8_to_1(Bit_5)/3, Bit_Multiplexer_8_to_1(Bit_6)/3, Bit_Multiplexer_8_to_1(Bit_7)/3
  Address_1(1b)/1 -> Bit_Multiplexer_8_to_1(Bit_5)/2, Bit_Multiplexer_8_to_1(Bit_0)/2, Bit_Multiplexer_8_to_1(Bit_1)/2, Bit_Multiplexer_8_to_1(Bit_2)/2, Bit_Multiplexer_8_to_1(Bit_3)/2, Bit_Multiplexer_8_to_1(Bit_4)/2, Bit_Multiplexer_8_to_1(Bit_6)/2, Bit_Multiplexer_8_to_1(Bit_7)/2
  Address_2(1b)/1 -> Bit_Multiplexer_8_to_1(Bit_0)/1, Bit_Multiplexer_8_to_1(Bit_1)/1, Bit_Multiplexer_8_to_1(Bit_2)/1, Bit_Multiplexer_8_to_1(Bit_3)/1, Bit_Multiplexer_8_to_1(Bit_4)/1, Bit_Multiplexer_8_to_1(Bit_5)/1, Bit_Multiplexer_8_to_1(Bit_6)/1, Bit_Multiplexer_8_to_1(Bit_7)/1
  Bit_Multiplexer_8_to_1(Bit_4)/1 -> Mux/4
  Bit_Multiplexer_8_to_1(Bit_5)/1 -> Mux/3
  Bit_Multiplexer_8_to_1(Bit_6)/1 -> Mux/2
  Bit_Multiplexer_8_to_1(Bit_7)/1 -> Mux/1
  Bit_Multiplexer_8_to_1(Bit_3)/1 -> Mux/5
  Bit_Multiplexer_8_to_1(Bit_2)/1 -> Mux/6
  Bit_Multiplexer_8_to_1(Bit_1)/1 -> Mux/7
  Bit_Multiplexer_8_to_1(Bit_0)/1 -> Mux/8
  Byte_0/8 -> Bit_0/8
  Byte_1/8 -> Bit_0/7
  Byte_2/8 -> Bit_0/6
  Byte_3/8 -> Bit_0/5
  Byte_4/8 -> Bit_0/4
  Byte_5/8 -> Bit_0/3
  Byte_6/8 -> Bit_0/2
  Byte_7/8 -> Bit_0/1
  Byte_0/7 -> Bit_1/8
  Byte_1/7 -> Bit_1/7
  Byte_2/7 -> Bit_1/6
  Byte_3/7 -> Bit_1/5
  Byte_4/7 -> Bit_1/4
  Byte_5/7 -> Bit_1/3
  Byte_6/7 -> Bit_1/2
  Byte_0/6 -> Bit_2/8
  Byte_1/6 -> Bit_2/7
  Byte_2/6 -> Bit_2/6
  Byte_3/6 -> Bit_2/5
  Byte_4/6 -> Bit_2/4
  Byte_5/6 -> Bit_2/3
  Byte_6/6 -> Bit_2/2
  Byte_7/6 -> Bit_2/1
  Byte_0/5 -> Bit_3/8
  Byte_1/5 -> Bit_3/7
  Byte_2/5 -> Bit_3/6
  Byte_3/5 -> Bit_3/5
  Byte_4/5 -> Bit_3/4
  Byte_5/5 -> Bit_3/3
  Byte_6/5 -> Bit_3/2
  Byte_7/5 -> Bit_3/1
  Byte_0/4 -> Bit_4/8
  Byte_1/4 -> Bit_4/7
  Byte_2/4 -> Bit_4/6
  Byte_3/4 -> Bit_4/5
  Byte_4/4 -> Bit_4/4
  Byte_5/4 -> Bit_4/3
  Byte_6/4 -> Bit_4/2
  Byte_7/4 -> Bit_4/1
  Byte_0/3 -> Bit_5/8
  Byte_1/3 -> Bit_5/7
  Byte_2/3 -> Bit_5/6
  Byte_3/3 -> Bit_5/5
  Byte_4/3 -> Bit_5/4
  Byte_5/3 -> Bit_5/3
  Byte_6/3 -> Bit_5/2
  Byte_7/3 -> Bit_5/1
  Byte_0/2 -> Bit_6/8
  Byte_1/2 -> Bit_6/7
  Byte_2/2 -> Bit_6/6
  Byte_3/2 -> Bit_6/5
  Byte_4/2 -> Bit_6/4
  Byte_5/2 -> Bit_6/3
  Byte_6/2 -> Bit_6/2
  Byte_7/2 -> Bit_6/1
  Byte_0/1 -> Bit_7/8
  Byte_1/1 -> Bit_7/7
  Byte_2/1 -> Bit_7/6
  Byte_3/1 -> Bit_7/5
  Byte_4/1 -> Bit_7/4
  Byte_5/1 -> Bit_7/3
  Byte_6/1 -> Bit_7/2
  Byte_7/1 -> Bit_7/1
  Integer to Bit Converter9/1 -> Byte_7/1
  Data_In_7(1B)/1 -> Integer to Bit Converter9/1
  Integer to Bit Converter10/1 -> Byte_6/1
  Data_In_6(1B)/1 -> Integer to Bit Converter10/1
  Integer to Bit Converter11/1 -> Byte_5/1
  Data_In_5(1B)/1 -> Integer to Bit Converter11/1
  Integer to Bit Converter12/1 -> Byte_4/1
  Data_In_4(1B)/1 -> Integer to Bit Converter12/1
  Integer to Bit Converter13/1 -> Byte_3/1
  Data_In_3(1B)/1 -> Integer to Bit Converter13/1
  Integer to Bit Converter14/1 -> Byte_2/1
  Data_In_2(1B)/1 -> Integer to Bit Converter14/1
  Integer to Bit Converter15/1 -> Byte_1/1
  Data_In_1(1B)/1 -> Integer to Bit Converter15/1
  Integer to Bit Converter16/1 -> Byte_0/1
  Data_In_0(1B)/1 -> Integer to Bit Converter16/1
  Demux/1 -> Bit_Multiplexer_8_to_1(Bit_7)/4
  Demux/2 -> Bit_Multiplexer_8_to_1(Bit_7)/5
  Demux/3 -> Bit_Multiplexer_8_to_1(Bit_7)/6
  Demux/4 -> Bit_Multiplexer_8_to_1(Bit_7)/7
  Demux/5 -> Bit_Multiplexer_8_to_1(Bit_7)/8
  Demux/6 -> Bit_Multiplexer_8_to_1(Bit_7)/9
  Demux/7 -> Bit_Multiplexer_8_to_1(Bit_7)/10
  Demux/8 -> Bit_Multiplexer_8_to_1(Bit_7)/11
  Demux1/1 -> Bit_Multiplexer_8_to_1(Bit_6)/4
  Demux1/2 -> Bit_Multiplexer_8_to_1(Bit_6)/5
  Demux1/3 -> Bit_Multiplexer_8_to_1(Bit_6)/6
  Demux1/4 -> Bit_Multiplexer_8_to_1(Bit_6)/7
  Demux1/5 -> Bit_Multiplexer_8_to_1(Bit_6)/8
  Demux1/6 -> Bit_Multiplexer_8_to_1(Bit_6)/9
  Demux1/7 -> Bit_Multiplexer_8_to_1(Bit_6)/10
  Demux1/8 -> Bit_Multiplexer_8_to_1(Bit_6)/11
  Demux2/1 -> Bit_Multiplexer_8_to_1(Bit_5)/4
  Demux2/2 -> Bit_Multiplexer_8_to_1(Bit_5)/5
  Demux2/3 -> Bit_Multiplexer_8_to_1(Bit_5)/6
  Demux2/4 -> Bit_Multiplexer_8_to_1(Bit_5)/7
  Demux2/5 -> Bit_Multiplexer_8_to_1(Bit_5)/8
  Demux2/6 -> Bit_Multiplexer_8_to_1(Bit_5)/9
  Demux2/7 -> Bit_Multiplexer_8_to_1(Bit_5)/10
  Demux2/8 -> Bit_Multiplexer_8_to_1(Bit_5)/11
  Demux3/1 -> Bit_Multiplexer_8_to_1(Bit_4)/4
  Demux3/2 -> Bit_Multiplexer_8_to_1(Bit_4)/5
  Demux3/3 -> Bit_Multiplexer_8_to_1(Bit_4)/6
  Demux3/4 -> Bit_Multiplexer_8_to_1(Bit_4)/7
  Demux3/5 -> Bit_Multiplexer_8_to_1(Bit_4)/8
  Demux3/6 -> Bit_Multiplexer_8_to_1(Bit_4)/9
  Demux3/7 -> Bit_Multiplexer_8_to_1(Bit_4)/10
  Demux3/8 -> Bit_Multiplexer_8_to_1(Bit_4)/11
  Demux4/1 -> Bit_Multiplexer_8_to_1(Bit_3)/4
  Demux4/2 -> Bit_Multiplexer_8_to_1(Bit_3)/5
  Demux4/3 -> Bit_Multiplexer_8_to_1(Bit_3)/6
  Demux4/4 -> Bit_Multiplexer_8_to_1(Bit_3)/7
  Demux4/5 -> Bit_Multiplexer_8_to_1(Bit_3)/8
  Demux4/6 -> Bit_Multiplexer_8_to_1(Bit_3)/9
  Demux4/7 -> Bit_Multiplexer_8_to_1(Bit_3)/10
  Demux4/8 -> Bit_Multiplexer_8_to_1(Bit_3)/11
  Demux5/1 -> Bit_Multiplexer_8_to_1(Bit_2)/4
  Demux5/2 -> Bit_Multiplexer_8_to_1(Bit_2)/5
  Demux5/3 -> Bit_Multiplexer_8_to_1(Bit_2)/6
  Demux5/4 -> Bit_Multiplexer_8_to_1(Bit_2)/7
  Demux5/5 -> Bit_Multiplexer_8_to_1(Bit_2)/8
  Demux5/6 -> Bit_Multiplexer_8_to_1(Bit_2)/9
  Demux5/7 -> Bit_Multiplexer_8_to_1(Bit_2)/10
  Demux5/8 -> Bit_Multiplexer_8_to_1(Bit_2)/11
  Demux6/1 -> Bit_Multiplexer_8_to_1(Bit_1)/4
  Demux6/2 -> Bit_Multiplexer_8_to_1(Bit_1)/5
  Demux6/3 -> Bit_Multiplexer_8_to_1(Bit_1)/6
  Demux6/4 -> Bit_Multiplexer_8_to_1(Bit_1)/7
  Demux6/5 -> Bit_Multiplexer_8_to_1(Bit_1)/8
  Demux6/6 -> Bit_Multiplexer_8_to_1(Bit_1)/9
  Demux6/7 -> Bit_Multiplexer_8_to_1(Bit_1)/10
  Demux6/8 -> Bit_Multiplexer_8_to_1(Bit_1)/11
  Demux7/1 -> Bit_Multiplexer_8_to_1(Bit_0)/4
  Demux7/2 -> Bit_Multiplexer_8_to_1(Bit_0)/5
  Demux7/3 -> Bit_Multiplexer_8_to_1(Bit_0)/6
  Demux7/4 -> Bit_Multiplexer_8_to_1(Bit_0)/7
  Demux7/5 -> Bit_Multiplexer_8_to_1(Bit_0)/8
  Demux7/6 -> Bit_Multiplexer_8_to_1(Bit_0)/9
  Demux7/7 -> Bit_Multiplexer_8_to_1(Bit_0)/10
  Demux7/8 -> Bit_Multiplexer_8_to_1(Bit_0)/11

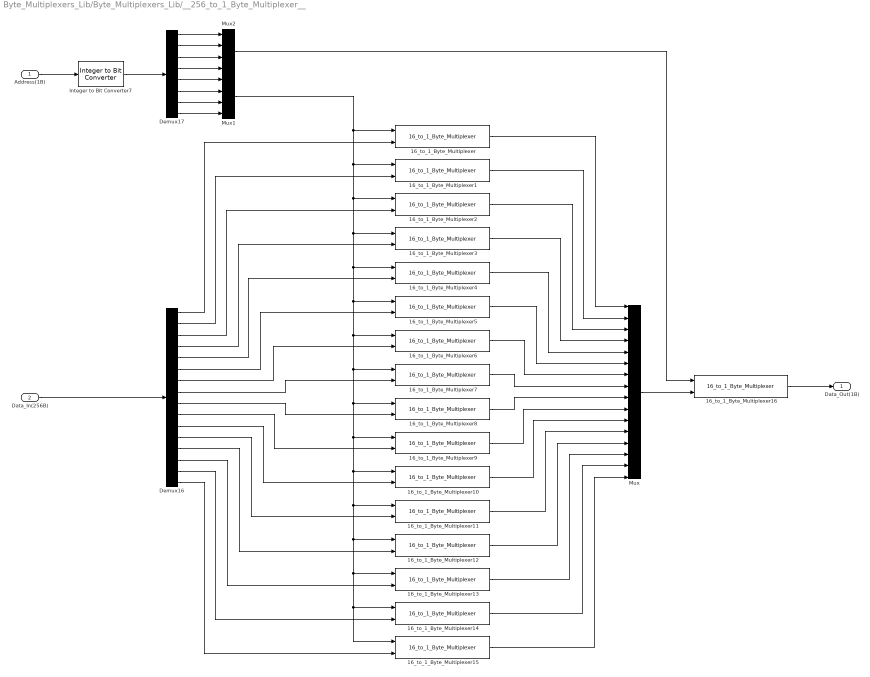
== system Byte_Multiplexers_Lib/Byte_Multiplexers_Lib/__256_to_1_Byte_Multiplexer__ ==
  Address(1B) : Inport
  Data_In(256B) : Inport  Port=2
  16_to_1_Byte_Multiplexer{,1..16} (17 alike) : Computer_Library/Multiplexers/16_to_1_Byte_Multiplexer
  Demux16 : Demux  Outputs=16
  Demux17 : Demux  Outputs=8
  Integer to Bit Converter7 : commutil2/Integer to Bit Converter  nbits=8  signedInputValues=Unsigned  bitOrder=MSB first  outDtype=boolean
  Mux : Mux  Inputs=16
  Mux1 : Mux
  Mux2 : Mux
  Data_Out(1B) : Outport
  wires:
  Address(1B)/1 -> Integer to Bit Converter7/1
  Integer to Bit Converter7/1 -> Demux17/1
  Mux2/1 -> 16_to_1_Byte_Multiplexer16/1
  Demux17/4 -> Mux2/4
  Demux17/3 -> Mux2/3
  Demux17/2 -> Mux2/2
  Demux17/1 -> Mux2/1
  Mux1/1 -> 16_to_1_Byte_Multiplexer/1, 16_to_1_Byte_Multiplexer2/1, 16_to_1_Byte_Multiplexer3/1, 16_to_1_Byte_Multiplexer4/1, 16_to_1_Byte_Multiplexer5/1, 16_to_1_Byte_Multiplexer6/1, 16_to_1_Byte_Multiplexer7/1, 16_to_1_Byte_Multiplexer8/1, 16_to_1_Byte_Multiplexer9/1, 16_to_1_Byte_Multiplexer10/1, 16_to_1_Byte_Multiplexer11/1, 16_to_1_Byte_Multiplexer12/1, 16_to_1_Byte_Multiplexer13/1, 16_to_1_Byte_Multiplexer14/1, 16_to_1_Byte_Multiplexer15/1, 16_to_1_Byte_Multiplexer1/1
  Demux17/8 -> Mux1/4
  Demux17/7 -> Mux1/3
  Demux17/6 -> Mux1/2
  Demux17/5 -> Mux1/1
  Demux16/16 -> 16_to_1_Byte_Multiplexer15/2
  Demux16/15 -> 16_to_1_Byte_Multiplexer14/2
  Demux16/14 -> 16_to_1_Byte_Multiplexer13/2
  Demux16/13 -> 16_to_1_Byte_Multiplexer12/2
  Demux16/12 -> 16_to_1_Byte_Multiplexer11/2
  Demux16/11 -> 16_to_1_Byte_Multiplexer10/2
  Demux16/10 -> 16_to_1_Byte_Multiplexer9/2
  Demux16/9 -> 16_to_1_Byte_Multiplexer8/2
  Demux16/8 -> 16_to_1_Byte_Multiplexer7/2
  Demux16/7 -> 16_to_1_Byte_Multiplexer6/2
  Demux16/6 -> 16_to_1_Byte_Multiplexer5/2
  Demux16/5 -> 16_to_1_Byte_Multiplexer4/2
  Demux16/4 -> 16_to_1_Byte_Multiplexer3/2
  Demux16/3 -> 16_to_1_Byte_Multiplexer2/2
  Demux16/2 -> 16_to_1_Byte_Multiplexer1/2
  Demux16/1 -> 16_to_1_Byte_Multiplexer/2
  16_to_1_Byte_Multiplexer16/1 -> Data_Out(1B)/1
  Data_In(256B)/1 -> Demux16/1
  Mux/1 -> 16_to_1_Byte_Multiplexer16/2
  16_to_1_Byte_Multiplexer15/1 -> Mux/16
  16_to_1_Byte_Multiplexer14/1 -> Mux/15
  16_to_1_Byte_Multiplexer13/1 -> Mux/14
  16_to_1_Byte_Multiplexer12/1 -> Mux/13
  16_to_1_Byte_Multiplexer11/1 -> Mux/12
  16_to_1_Byte_Multiplexer10/1 -> Mux/11
  16_to_1_Byte_Multiplexer9/1 -> Mux/10
  16_to_1_Byte_Multiplexer8/1 -> Mux/9
  16_to_1_Byte_Multiplexer7/1 -> Mux/8
  16_to_1_Byte_Multiplexer6/1 -> Mux/7
  16_to_1_Byte_Multiplexer5/1 -> Mux/6
  16_to_1_Byte_Multiplexer4/1 -> Mux/5
  16_to_1_Byte_Multiplexer3/1 -> Mux/4
  16_to_1_Byte_Multiplexer2/1 -> Mux/3
  16_to_1_Byte_Multiplexer1/1 -> Mux/2
  16_to_1_Byte_Multiplexer/1 -> Mux/1
